simulink model "Tema3_Slink"  (R2014a)
settings: Solver=ode45  StartTime=0.0  StopTime=10.0  RelTol=1e-3
values from neighbouring files (symbols this model uses):
  A = 9    [Tema3.m]    (also in Tema4.m = 0.1)
  d2 = 4    [Tema2.m]    (also in Tema3.m = 0.0055; Tema4.m = 0.2; Tema7.m = 0.2)
libraries: cstblocks x2, simulink x2
settings Model: Creator=giova  LastModifiedBy=giova

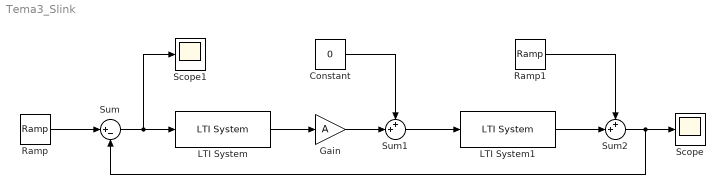
== system Tema3_Slink ==
  Constant : Constant  Value=0
  Gain : Gain  Gain=A
  LTI System : cstblocks/LTI System  sys=C  IC=[]
  LTI System1 : cstblocks/LTI System  sys=F1  IC=[]
  Ramp : simulink/Sources/Ramp  slope=0  start=0  X0=0
  Ramp1 : simulink/Sources/Ramp  slope=d2  start=0  X0=0
  Scope : Scope
  Scope1 : Scope
  Sum : Sum  Inputs=|+-
  Sum1 : Sum  Inputs=++|
  Sum2 : Sum  Inputs=++|
  wires:
  Gain/1 -> Sum1/2
  Sum1/1 -> LTI System1/1
  LTI System/1 -> Gain/1
  LTI System1/1 -> Sum2/2
  Sum2/1 -> Sum/2, Scope/1
  Sum/1 -> Scope1/1, LTI System/1
  Ramp/1 -> Sum/1
  Constant/1 -> Sum1/1
  Ramp1/1 -> Sum2/1
